simulink model "motor_model_updated2"  (R2020a)
settings: Solver=ode1  StartTime=0.0  StopTime=inf  FixedStep=0.0001  RelTol=1e-3  EnableMultiTasking=on
libraries: arduinolib x5, simulink x2
settings Model: SimulationMode=external  SILPILModeSetting=veronly  ExtModeTrigDuration=2  Creator=Ninad  LastModifiedBy=Jeremy
settings DataIOCC: LimitDataPoints=on  SaveFormat=Array  SignalLoggingSaveFormat=ModelDataLogs  ReturnWorkspaceOutputs=off
settings OptimizationCC: BlockReduction=off  EnhancedBackFolding=on  PassReuseOutputArgsAs=Individual arguments  ExpressionDepthLimit=2147483647  ZeroExternalMemoryAtStartup=off  ZeroInternalMemoryAtStartup=off  MaxStackSize=64  OptimizeBlockOrder=speed  DifferentSizesBufferReuse=on  OptimizationCustomize=off  EfficientTunableParamExpr=on
settings DebuggingCC: UnderspecifiedInitializationDetection=Classic  MergeDetectMultiDrivingBlocksExec=none  SolverPrmCheckMsg=warning  ParameterTunabilityLossMsg=error  FcnCallInpInsideContextMsg=warning  StateNameClashWarn=warning  SFUnexpectedBacktrackingDiag=warning  SFNoUnconditionalDefaultTransitionDiag=warning  SFExecutionAtInitializationDiag=none  ArithmeticOperatorsInVariantConditions=warning
settings HardwareCC: ProdBitPerInt=16  ProdBitPerPointer=16  ProdBitPerSizeT=16  ProdBitPerPtrDiffT=16  ProdLargestAtomicFloat=None  ProdWordSize=8  ProdHWDeviceType=Atmel->AVR  UseEmbeddedCoderFeatures=off
settings ModelReferenceCC: PropagateSignalLabelsOutOfModel=off
settings SFSimCC: SimUseLocalCustomCode=off  MATLABDynamicMemAlloc=off  CustomCodeUndefinedFunction=UseInterfaceOnly
settings RTWCC: SystemTargetFile=ert.tlc  HardwareBoard=Arduino Mega 2560  TLCOptions=-aInlineSetEventsForThisBaseRateFcn=TLC_FALSE -aSuppressMultiTaskScheduler=TLC_FALSE -aRateBasedStepFcn=1  TemplateMakefile=ert_default_tmf  RTWUseLocalCustomCode=off  Toolchain=Arduino AVR  BuildConfiguration=Faster Runs  CodeExecutionProfiling=on
settings CodeAppCC: ForceParamTrailComments=on  IgnoreCustomStorageClasses=off  OperatorAnnotations=on  SimulinkDataObjDesc=on  SFDataObjDesc=on  InsertBlockDesc=on
settings ERTTargetCC: SupportContinuousTime=on  SupportNonInlinedSFcns=on  SupportVariableSizeSignals=on  ExtModeStaticAllocSize=2048
settings ConfigComp: CovMetricSettings=dw  CovHtmlReporting=on  CovSaveCumulativeToWorkspaceVar=on  CovSaveSingleToWorkspaceVar=on  CovExternalEMLEnable=off  CovSFcnEnable=off

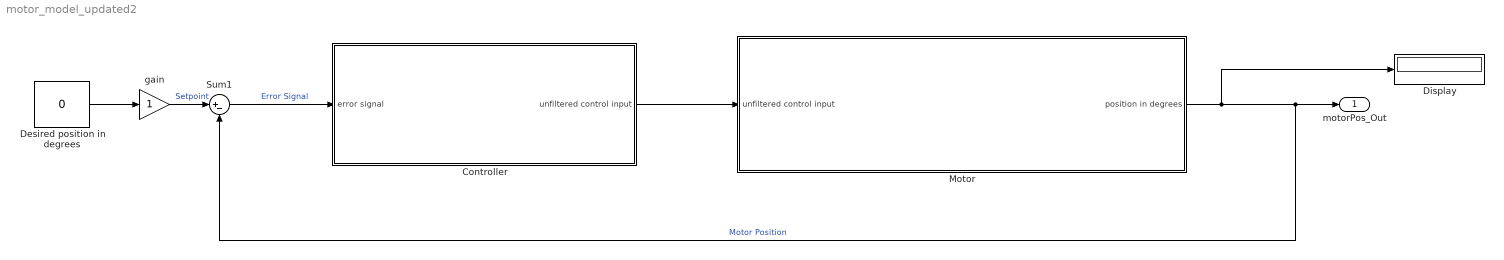
== system motor_model_updated2 ==
  Controller : Subsystem
  Desired position in degrees : Constant  Value=0
  Display : Display
  Motor : Subsystem
  Sum1 : Sum  Inputs=|+-
  gain : Gain
  motorPos_Out : Outport  VectorParamsAs1DForOutWhenUnconnected=off
  wires:
  gain/1 -> Sum1/1  "Setpoint"
  Desired position in degrees/1 -> gain/1
  Motor/1(position in degrees) -> Display/1, Sum1/2, motorPos_Out/1  "Motor Position"
  Controller/1(unfiltered control input) -> Motor/1(unfiltered control input)
  Sum1/1 -> Controller/1(error signal)  "Error Signal"

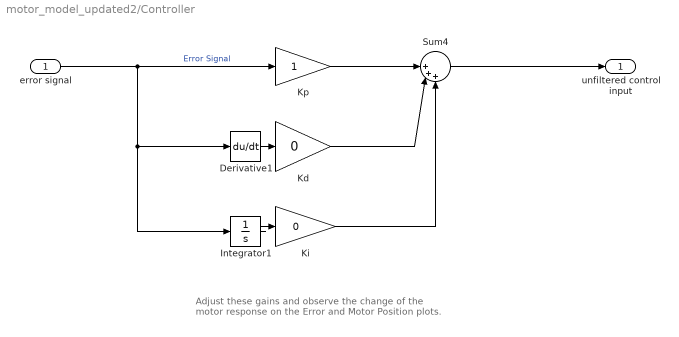
== system motor_model_updated2/Controller ==
  note: Adjust these gains and observe the change of the
      | motor response on the Error and Motor Position
      | plots.
  error signal : Inport
  Derivative1 : Derivative
  Integrator1 : Integrator
  Kd : Gain  Gain=0
  Ki : Gain  Gain=0
  Kp : Gain
  Sum4 : Sum  Inputs=||+++
  unfiltered control input : Outport
  wires:
  Kd/1 -> Sum4/2
  Integrator1/1 -> Ki/1
  Ki/1 -> Sum4/3
  Derivative1/1 -> Kd/1
  error signal/1 -> Derivative1/1, Integrator1/1, Kp/1  "Error Signal"
  Kp/1 -> Sum4/1
  Sum4/1 -> unfiltered control input/1

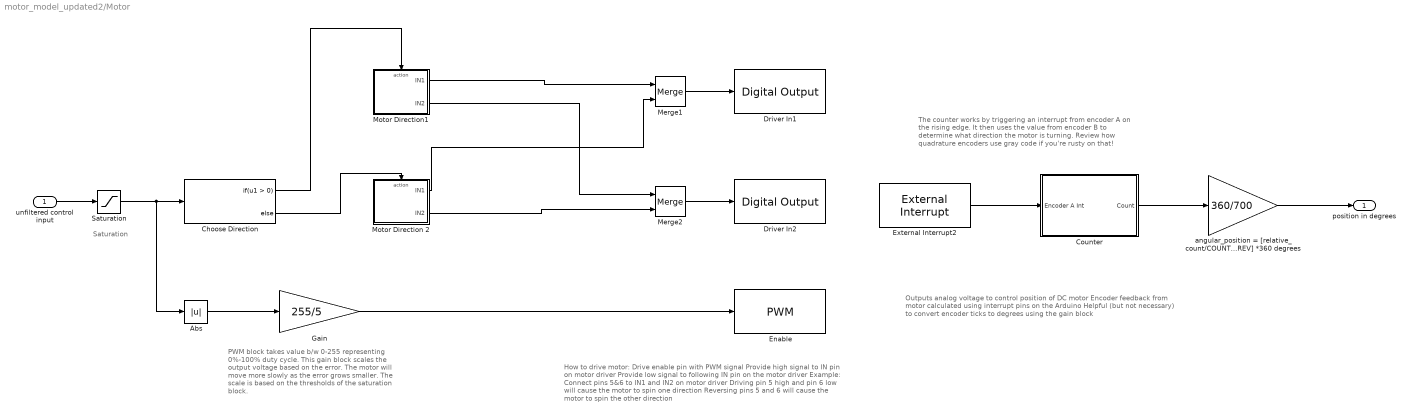
== system motor_model_updated2/Motor ==
  note: The counter works by triggering an interrupt from encoder A
      | on the rising edge. It then uses the value from encoder B to
      | determine what direction the motor is turning. Review how
      | quadrature encoders use gray code if you're rusty on that!
  note: PWM block takes value b/w 0-255 representing
      | 0%-100% duty cycle. This gain block scales the
      | output voltage based on the error. The motor will
      | move more slowly as the error grows
      | smaller. The scale is based on the thresholds
      | of the saturation block.
  note: Outputs analog voltage to control position of DC motor
      |
      | Encoder feedback from motor calculated using interrupt pins on the Arduino
      |
      | Helpful (but not necessary) to convert encoder ticks to degrees using the
      | gain block
  note: Saturation
  note: How to drive motor:
      | Drive enable pin with PWM signal
      | Provide high signal to IN pin on motor driver
      | Provide low signal to following IN pin on the motor driver
      |
      | Example:
      | Connect pins 5&6 to IN1 and IN2 on motor driver
      | Driving pin 5 high and pin 6 low will cause the motor to spin one direction
      | Reversing pins 5 and 6 will cause the motor to spin the other direction
  unfiltered control input : Inport
  Abs : Abs
  Choose Direction : If
  Counter : Subsystem
  Driver In1 : arduinolib/Digital Output  pinNumber=30  Direction=output  blockPlatform=arduino
  Driver In2 : arduinolib/Digital Output  pinNumber=31  Direction=output  blockPlatform=arduino
  Enable : arduinolib/PWM  pinNumber=5  frequencyType=Default  desiredFrequency=490.2  achievableFrequency=490.2
  External Interrupt2 : arduinolib/External Interrupt  Pin=2  PullUp=on  Mode=RISING  InterruptSimulationInput=off
      settings: SourceProductBaseCode=ARDUINO
  Gain : Gain  Gain=255/5
  Merge1 : Merge
  Merge2 : Merge
  Motor Direction 2 : Subsystem  TreatAsAtomicUnit=on
  Motor Direction1 : Subsystem  TreatAsAtomicUnit=on
  Saturation : Saturate  UpperLimit=5  LowerLimit=-5
  angular_position = [relative_count/COUNTS_PER_REV] *360 degrees : Gain  Gain=360/700
  position in degrees : Outport  VectorParamsAs1DForOutWhenUnconnected=off
  wires:
  angular_position = [relative_count/COUNTS_PER_REV] *360 degrees/1 -> position in degrees/1
  unfiltered control input/1 -> Saturation/1
  Counter/1(Count) -> angular_position = [relative_count/COUNTS_PER_REV] *360 degrees/1
  Saturation/1 -> Abs/1, Choose Direction/1
  Choose Direction/1 -> Motor Direction1/Action
  Choose Direction/2 -> Motor Direction 2/Action
  Motor Direction1/1(IN1) -> Merge1/1
  Motor Direction 2/1(IN1) -> Merge1/2
  Motor Direction1/2(IN2) -> Merge2/1
  Motor Direction 2/2(IN2) -> Merge2/2
  Abs/1 -> Gain/1
  Gain/1 -> Enable/1
  Merge1/1 -> Driver In1/1
  Merge2/1 -> Driver In2/1
  External Interrupt2/1 -> Counter/1(Encoder A Int)

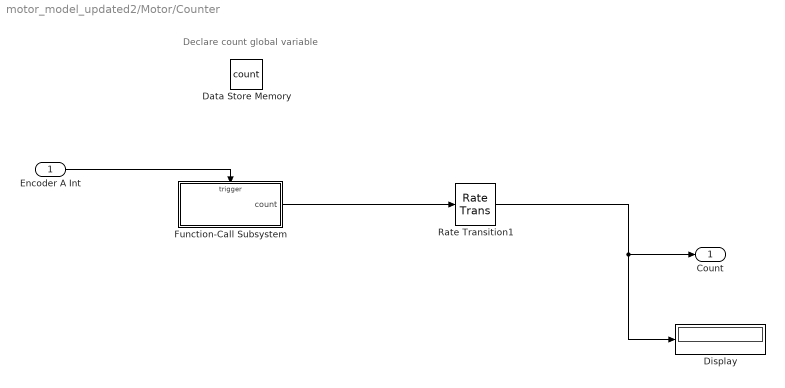
== system motor_model_updated2/Motor/Counter ==
  note: Declare count global variable
  Encoder A Int : Inport
  Data Store Memory : DataStoreMemory  DataStoreName=count  ReadBeforeWriteMsg=warning  WriteAfterWriteMsg=warning  WriteAfterReadMsg=warning  ShowAdditionalParam=off
  Display : Display
  Function-Call Subsystem : Subsystem  TreatAsAtomicUnit=on
  Rate Transition1 : RateTransition  Deterministic=off
  Count : Outport
  wires:
  Encoder A Int/1 -> Function-Call Subsystem/Trigger
  Function-Call Subsystem/1(count) -> Rate Transition1/1
  Rate Transition1/1 -> Display/1, Count/1

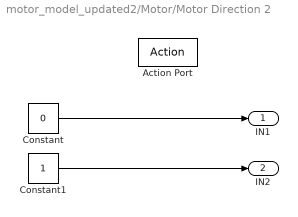
== system motor_model_updated2/Motor/Motor Direction 2 ==
  Action Port : ActionPort  ActionPortLabel=else
  Constant : Constant  Value=0
  Constant1 : Constant
  IN1 : Outport
  IN2 : Outport  Port=2
  wires:
  Constant/1 -> IN1/1
  Constant1/1 -> IN2/1

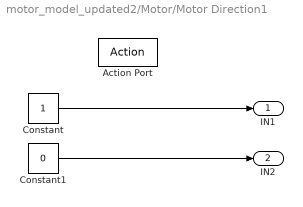
== system motor_model_updated2/Motor/Motor Direction1 ==
  Action Port : ActionPort  ActionPortLabel=if(u1 > 0)
  Constant : Constant
  Constant1 : Constant  Value=0
  IN1 : Outport
  IN2 : Outport  Port=2
  wires:
  Constant/1 -> IN1/1
  Constant1/1 -> IN2/1

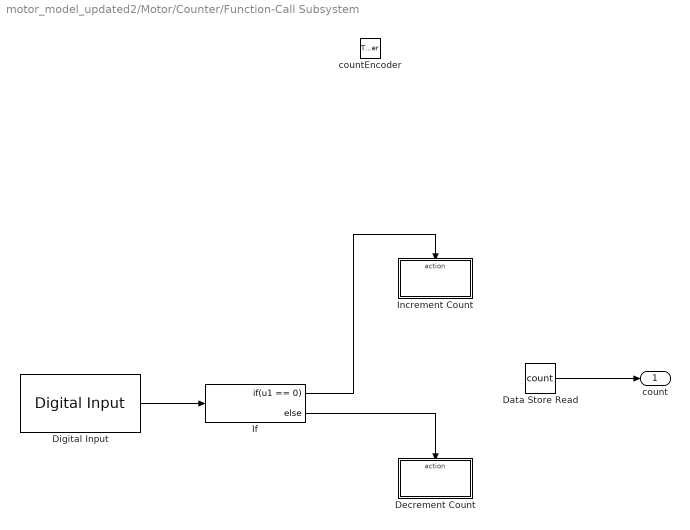
== system motor_model_updated2/Motor/Counter/Function-Call Subsystem ==
  countEncoder : TriggerPort  TriggerType=function-call  VariantControl=Variant
  Data Store Read : DataStoreRead  DataStoreName=count
  Decrement Count : Subsystem  TreatAsAtomicUnit=on
  Digital Input : arduinolib/Digital Input  pinNumber=3  Direction=input  SampleTime=-1  blockPlatform=arduino
  If : If  IfExpression=u1 == 0
  Increment Count : Subsystem  TreatAsAtomicUnit=on
  count : Outport
  wires:
  If/2 -> Decrement Count/Action
  If/1 -> Increment Count/Action
  Data Store Read/1 -> count/1
  Digital Input/1 -> If/1

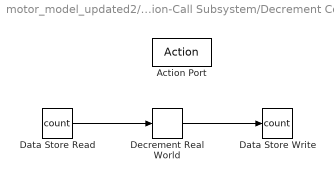
== system motor_model_updated2/Motor/Counter/Function-Call Subsystem/Decrement Count ==
  Action Port : ActionPort  ActionPortLabel=else
  Data Store Read : DataStoreRead  DataStoreName=count
  Data Store Write : DataStoreWrite  DataStoreName=count
  Decrement Real World : simulink/Additional Math & Discrete/Additional Math: Increment - Decrement/Decrement Real World
      settings: SourceProductBaseCode=SL
  wires:
  Data Store Read/1 -> Decrement Real World/1
  Decrement Real World/1 -> Data Store Write/1

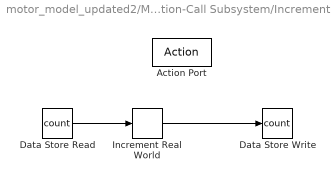
== system motor_model_updated2/Motor/Counter/Function-Call Subsystem/Increment Count ==
  Action Port : ActionPort  ActionPortLabel=if(u1 == 0)
  Data Store Read : DataStoreRead  DataStoreName=count
  Data Store Write : DataStoreWrite  DataStoreName=count
  Increment Real World : simulink/Additional Math & Discrete/Additional Math: Increment - Decrement/Increment Real World
      settings: SourceProductBaseCode=SL
  wires:
  Data Store Read/1 -> Increment Real World/1
  Increment Real World/1 -> Data Store Write/1
